simulink library "actuator_lib"  (Simulink 7.2)
settings: Solver=ode45  SolverMode=SingleTasking  StartTime=0.0  StopTime=10.0  RelTol=1e-3
libraries: actuator_T2_lib x2, simulink x1
settings Model: Creator=amurch  LastModifiedBy=la1032aw  ExtModeAutoUpdateStatusClock=off

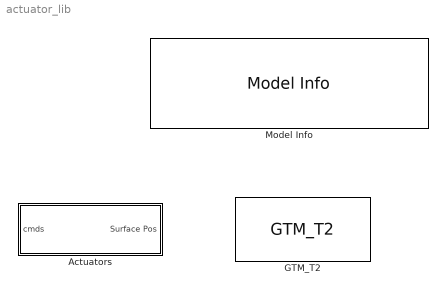
== system actuator_lib ==
  Actuators : Subsystem  BlockChoice=GTM_T2
      settings: TemplateBlock=self  MemberBlocks=GTM_T2
  GTM_T2 : actuator_T2_lib/GTM_T2  SystemSampleTime=-1
  Model Info : simulink/Model-Wide Utilities/Model Info  SystemSampleTime=-1  InitialBlockCM=None  BlockCM=None  Frame=on  DisplayStringWithTags=|  HorizontalTextAlignment=Center  LeftAlignmentValue=0.5  SourceBlockDiagram=actuator_lib  TagMaxNumber=20
      | Actuator Library
      | %<ModelVersion>
      | Las modified by %<LastModifiedBy> on %<LastModificationDate>

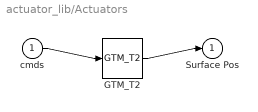
== system actuator_lib/Actuators ==
  cmds : Inport  OutDataType=sfix(16)  OutScaling=2^0
  GTM_T2 : actuator_T2_lib/GTM_T2  SystemSampleTime=-1
  Surface Pos : Outport  OutDataType=sfix(16)  OutScaling=2^0
  wires:
  cmds/1 -> GTM_T2/1
  GTM_T2/1 -> Surface Pos/1
